simulink model "simple_single_ph_PLL"  (R2020b)
settings: Solver=VariableStepAuto  StartTime=0.0  StopTime=30  MaxStep=1e-5  MinStep=1e-7
libraries: simulink x4, eeStairGenerator x3
settings Model: Creator=Kasper Laustsen  LastModifiedBy=martin

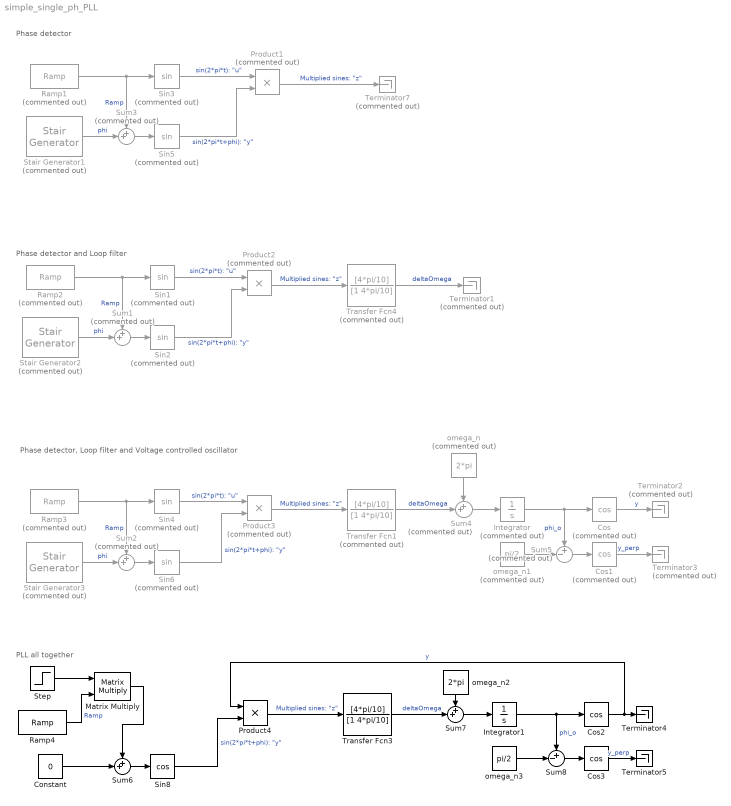
== system simple_single_ph_PLL ==
  note: Phase detector
  note: Phase detector and Loop filter
  note: Phase detector, Loop filter and Voltage controlled oscillator
  note: PLL all together
  Constant : Constant  Value=0
  Cos : Trigonometry  Commented=on  Operator=cos
  Cos1 : Trigonometry  Commented=on  Operator=cos
  Cos2 : Trigonometry  Operator=cos
  Cos3 : Trigonometry  Operator=cos
  Integrator : Integrator  Commented=on
  Integrator1 : Integrator
  Matrix Multiply : Product  Multiplication=Matrix(*)
  Product1 : Product  Commented=on
  Product2 : Product  Commented=on
  Product3 : Product  Commented=on
  Product4 : Product
  Ramp1 : simulink/Sources/Ramp  Commented=on  slope=2*pi  start=0  InitialOutput=0
  Ramp2 : simulink/Sources/Ramp  Commented=on  slope=2*pi  start=0  InitialOutput=0
  Ramp3 : simulink/Sources/Ramp  Commented=on  slope=2*pi  start=0  InitialOutput=0
  Ramp4 : simulink/Sources/Ramp  slope=2*pi  start=0  InitialOutput=0
  Sin{1..6} (6 alike) : Trigonometry  Commented=on
  Sin8 : Trigonometry  Operator=cos
  Stair Generator1 : eeStairGenerator/Stair Generator  Commented=on  LabelModeActiveChoice=Discrete  TimeInput=[0 20 40 60 80 100 120 140 160 180]  AmplitudeInput=[-2*pi -(7/4)*pi -(6/4)*pi -(5/4)*pi -(4/4)*pi -(3/4)*pi -(2/4)*pi -(1/4)*pi 0 0]  SampleTime=1e-3  RepeatPattern=on  OutDataTypeStr=double
      settings: SourceProductBaseCode=PS
  Stair Generator2 : eeStairGenerator/Stair Generator  Commented=on  LabelModeActiveChoice=Discrete  TimeInput=[0 20 40 60 80 100 120 140 160 180]  AmplitudeInput=[-2*pi -(7/4)*pi -(6/4)*pi -(5/4)*pi -(4/4)*pi -(3/4)*pi -(2/4)*pi -(1/4)*pi 0 0]  SampleTime=1e-3  RepeatPattern=on  OutDataTypeStr=double
      settings: SourceProductBaseCode=PS
  Stair Generator3 : eeStairGenerator/Stair Generator  Commented=on  LabelModeActiveChoice=Discrete  TimeInput=[0 20 40 60 80 100 120 140 160 180]  AmplitudeInput=[-2*pi -(7/4)*pi -(6/4)*pi -(5/4)*pi -(4/4)*pi -(3/4)*pi -(2/4)*pi -(1/4)*pi 0 0]  SampleTime=1e-3  RepeatPattern=on  OutDataTypeStr=double
      settings: SourceProductBaseCode=PS
  Step : Step  Time=2  Before=1  SampleTime=0
  Sum{1..4} (4 alike) : Sum  Commented=on  Inputs=++|
  Sum5 : Sum  Commented=on  Inputs=+-|
  Sum6 : Sum  Inputs=++|
  Sum7 : Sum  Inputs=++|
  Sum8 : Sum  Inputs=+-|
  Terminator{1..3,7} (4 alike) : Terminator  Commented=on
  Terminator4 : Terminator
  Terminator5 : Terminator
  Transfer Fcn1 : TransferFcn  Commented=on  Numerator=[4*pi/10]  Denominator=[1 4*pi/10]
  Transfer Fcn3 : TransferFcn  Numerator=[4*pi/10]  Denominator=[1 4*pi/10]
  Transfer Fcn4 : TransferFcn  Commented=on  Numerator=[4*pi/10]  Denominator=[1 4*pi/10]
  omega_n : Constant  Commented=on  Value=2*pi
  omega_n1 : Constant  Commented=on  Value=pi/2
  omega_n2 : Constant  Value=2*pi
  omega_n3 : Constant  Value=pi/2
  wires:
  Product1/1 -> Terminator7/1  "Multiplied sines: \"z\""
  Sum3/1 -> Sin5/1
  Stair Generator1/1 -> Sum3/2  "phi"
  Sin5/1 -> Product1/2  "sin(2*pi*t+phi): \"y\""
  Sin3/1 -> Product1/1  "sin(2*pi*t): \"u\""
  Ramp1/1 -> Sin3/1, Sum3/1  "Ramp"
  Stair Generator2/1 -> Sum1/2  "phi"
  Ramp2/1 -> Sin1/1, Sum1/1  "Ramp"
  Product2/1 -> Transfer Fcn4/1  "Multiplied sines: \"z\""
  Sin2/1 -> Product2/2  "sin(2*pi*t+phi): \"y\""
  Sin1/1 -> Product2/1  "sin(2*pi*t): \"u\""
  Sum1/1 -> Sin2/1
  Transfer Fcn4/1 -> Terminator1/1  "deltaOmega"
  Sum2/1 -> Sin6/1
  Sin4/1 -> Product3/1  "sin(2*pi*t): \"u\""
  Sin6/1 -> Product3/2  "sin(2*pi*t+phi): \"y\""
  Stair Generator3/1 -> Sum2/2  "phi"
  Ramp3/1 -> Sin4/1, Sum2/1  "Ramp"
  Product3/1 -> Transfer Fcn1/1  "Multiplied sines: \"z\""
  Transfer Fcn1/1 -> Sum4/2  "deltaOmega"
  omega_n/1 -> Sum4/1
  Sum4/1 -> Integrator/1
  Integrator/1 -> Sum5/1, Cos/1  "phi_o"
  omega_n1/1 -> Sum5/2
  Sum5/1 -> Cos1/1
  Cos/1 -> Terminator2/1  "y"
  Cos1/1 -> Terminator3/1  "y_perp"
  Sum7/1 -> Integrator1/1
  Transfer Fcn3/1 -> Sum7/2  "deltaOmega"
  Sin8/1 -> Product4/2  "sin(2*pi*t+phi): \"y\""
  Cos2/1 -> Product4/1, Terminator4/1  "y"
  Sum8/1 -> Cos3/1
  Sum6/1 -> Sin8/1
  Cos3/1 -> Terminator5/1  "y_perp"
  Product4/1 -> Transfer Fcn3/1  "Multiplied sines: \"z\""
  Ramp4/1 -> Matrix Multiply/2  "Ramp"
  Integrator1/1 -> Sum8/1, Cos2/1  "phi_o"
  omega_n2/1 -> Sum7/1
  omega_n3/1 -> Sum8/2
  Step/1 -> Matrix Multiply/1
  Matrix Multiply/1 -> Sum6/1
  Constant/1 -> Sum6/2
